simulink model "system_simulation"  (R2018b)
settings: Solver=VariableStepAuto  StartTime=0.0  StopTime=10.0  RelTol=1e-3
undefined symbols (not defined in the file or in its folder): Ts
settings Model: Creator=Alireza  LastModifiedBy=Alireza

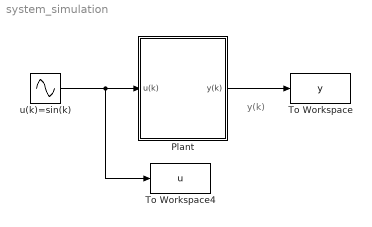
== system system_simulation ==
  note: y(k)
  Plant : Subsystem
  To Workspace : ToWorkspace  VariableName=y  SampleTime=Ts
      settings: Save2DSignal=2-D array (concatenate along first dimension)
  To Workspace4 : ToWorkspace  VariableName=u  SampleTime=Ts
      settings: Save2DSignal=2-D array (concatenate along first dimension)
  u(k)=sin(k) : Sin  SampleTime=Ts
  wires:
  Plant/1(y(k)) -> To Workspace/1
  u(k)=sin(k)/1 -> To Workspace4/1, Plant/1(u(k))

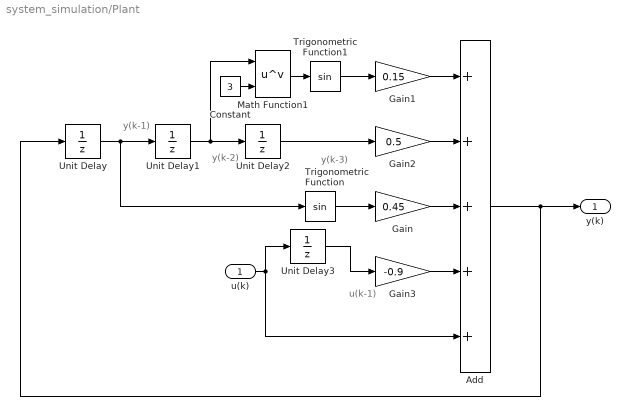
== system system_simulation/Plant ==
  note: y(k-1)
  note: y(k-2)
  note: y(k-3)
  note: u(k-1)
  u(k) : Inport
  Add : Sum  Inputs=+++++
  Constant : Constant  Value=3
  Gain : Gain  Gain=0.45
  Gain1 : Gain  Gain=0.15
  Gain2 : Gain  Gain=0.5
  Gain3 : Gain  Gain=-0.9
  Math Function1 : Math  Operator=pow  SaturateOnIntegerOverflow=on
  Trigonometric Function : Trigonometry
  Trigonometric Function1 : Trigonometry
  Unit Delay{,1..3} (4 alike) : UnitDelay  SampleTime=Ts
  y(k) : Outport
  wires:
  Unit Delay/1 -> Unit Delay1/1, Trigonometric Function/1
  Unit Delay1/1 -> Unit Delay2/1, Math Function1/1
  Trigonometric Function/1 -> Gain/1
  Math Function1/1 -> Trigonometric Function1/1
  Trigonometric Function1/1 -> Gain1/1
  Unit Delay2/1 -> Gain2/1
  Unit Delay3/1 -> Gain3/1
  Add/1 -> y(k)/1, Unit Delay/1
  Gain1/1 -> Add/1
  Gain2/1 -> Add/2
  Gain/1 -> Add/3
  Gain3/1 -> Add/4
  u(k)/1 -> Unit Delay3/1, Add/5
  Constant/1 -> Math Function1/2
